simulink model "move2"  (Simulink 7.5)
settings: Solver=VariableStepDiscrete  StartTime=0.0  StopTime=inf  RelTol=1e-3
libraries: simulink x2, vrlib x2
settings Model: Creator=falter  LastModifiedBy=falter
settings SolverCC: MaxConsecutiveZCs=10

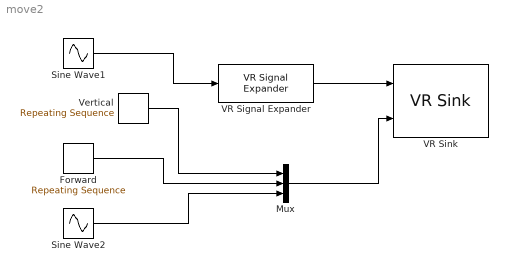
== system move2 ==
  Forward : simulink/Sources/Repeating Sequence  SystemSampleTime=-1  rep_seq_t=[0 32]  rep_seq_y=[2 2]
  Mux : Mux  Inputs=3
  Sine Wave1 : Sin  Amplitude=10  Bias=0  Frequency=0.03  Phase=0  Samples=10  SampleTime=0  Offset=0
  Sine Wave2 : Sin  Amplitude=10  Bias=0  Frequency=0.03  Phase=0  Samples=10  SampleTime=0  Offset=0
  VR Signal Expander : vrlib/VR Signal Expander  SystemSampleTime=-1  outwidth=4  outidx=[2 4]
  VR Sink : vrlib/VR Sink  InstantiateOnLoad=on  SampleTime=0.1  ViewEnable=on  RemoteChange=off  RemoteView=off  FieldsWritten=Falter.rotation.4.1.1.double#Falter.translation.3.1.1.double  WorldFileName=room.wrl  WorldDescription=Falter in a room  AutoView=on  VideoDimensions=[]
  Vertical : simulink/Sources/Repeating Sequence  SystemSampleTime=-1  rep_seq_t=[0 2 4 8 16 32]  rep_seq_y=[0 0 0 0 0 0]
  wires:
  VR Signal Expander/1 -> VR Sink/1
  Mux/1 -> VR Sink/2
  Vertical/1 -> Mux/1
  Forward/1 -> Mux/2
  Sine Wave1/1 -> VR Signal Expander/1
  Sine Wave2/1 -> Mux/3
